simulink model "Implementation_old"  (R2018a)
settings: Solver=ode3  StartTime=0.0  StopTime=50  RelTol=1e-3  EnableMultiTasking=on
values from neighbouring files (symbols this model uses):
  A = [3.3545 -4.3521 2.6058 -0.6082; 1 0 0 0; 0 1 0 0; 0 0 1 0]    [LQGm.m]    (also in Testes_planta.m)
  B = [1;0;0;0]    [LQGm.m]    (also in Testes_planta.m)
  C = [-0.0657 0.1152 0 0]    [LQGm.m]    (also in Testes_planta.m)
  ExtensometerGain = -4.49    [Testes_planta.m]
  Nbar = Nu+K*Nx    [LQGm.m]    (also in Testes_planta.m)
  PotentiometerGain = 33.79    [Testes_planta.m]
undefined symbols (not defined in the file or in its folder): DiscIntNeverNeededParam, K, M, MIO, National_Instruments, PCI
libraries: sldrtlib x2
settings Model: SimulationMode=external  ExtModeTrigDuration=20000  Creator=Alunos  LastModifiedBy=joaj
settings DataIOCC: LimitDataPoints=on  SaveFormat=Array
settings DebuggingCC: LibraryContextMissingDiagnostic=warning  SFUnexpectedBacktrackingDiag=warning  SFNoUnconditionalDefaultTransitionDiag=warning  SFExecutionAtInitializationDiag=none
settings HardwareCC: TargetIntDivRoundTo=Zero  TargetEndianess=LittleEndian  TargetHWDeviceType=Intel->x86/Pentium
settings ModelReferenceCC: PropagateSignalLabelsOutOfModel=off
settings RTWCC: SystemTargetFile=sldrt.tlc  TemplateMakefile=sldrt.tmf  Description=Simulink Desktop Real-Time  RTWCompilerOptimization=on
settings CodeAppCC: MaxIdLength=95  StateflowObjectComments=on
settings SimulinkDesktopRealTimeCC: TargetPreCompLibLocation=C:\Program Files\MATLAB\R2018b\toolbox\sldrt\lib\win64  TargetLangStandard=C89/C90 (ANSI)  SupportVariableSizeSignals=off
settings ConfigComp: CovMetricSettings=dw  CovHtmlReporting=on  CovSaveCumulativeToWorkspaceVar=on  CovSaveSingleToWorkspaceVar=on  CovExternalEMLEnable=off

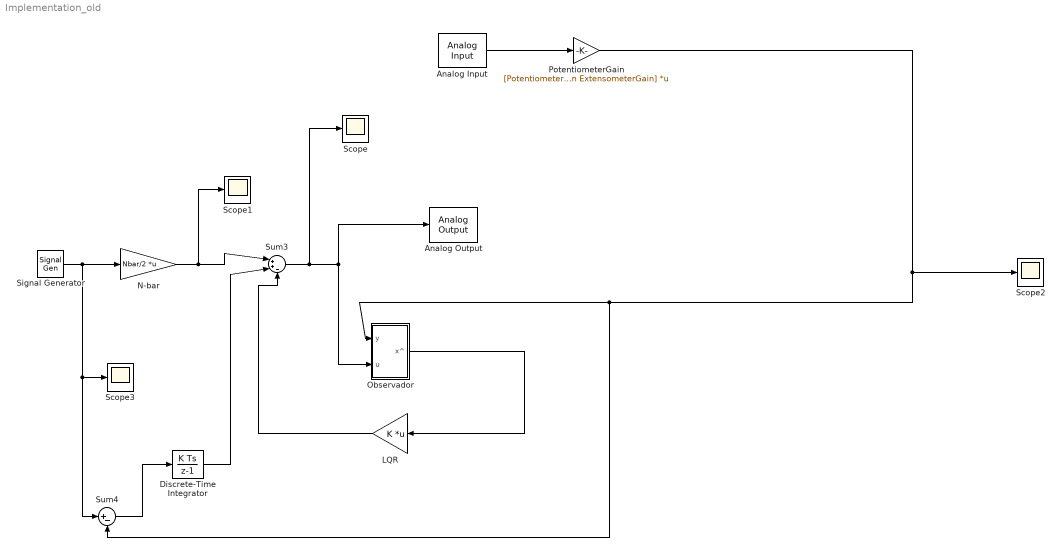
== system Implementation_old ==
  Analog Input : sldrtlib/Analog Input  SampleTime=0.02  MaxMissedTicks=10  ShowMissedTicks=off  YieldWhenWaiting=off  DrvName=National_Instruments/PCI-MIO-16E-4  DrvAddress=4294967295  DrvOptions=[0 0 0 0 0 0]  Channels=[1 2]  RangeMode=1  VoltRange=1  DataType=1
      settings: AttributesFormatString=National Instruments\nPCI-MIO-16E-4 [auto]  SourceProductName=Simulink Desktop Real-Time
  Analog Output : sldrtlib/Analog Output  SampleTime=0.02  MaxMissedTicks=10  ShowMissedTicks=off  YieldWhenWaiting=off  DrvName=National_Instruments/PCI-MIO-16E-4  DrvAddress=4294967295  DrvOptions=[0 0 0 0 0 0]  Channels=1  RangeMode=1  VoltRange=1  InitialValue=0  FinalValue=0
      settings: AttributesFormatString=National Instruments\nPCI-MIO-16E-4 [auto]  SourceProductName=Simulink Desktop Real-Time
  Discrete-Time Integrator : DiscreteIntegrator  gainval=1e-2  ICPrevOutput=DiscIntNeverNeededParam  ICPrevScaledInput=DiscIntNeverNeededParam
  LQR : Gain  Gain=K  Multiplication=Matrix(K*u)
  N-bar : Gain  Gain=Nbar/2  Multiplication=Matrix(K*u)
  Observador : Subsystem
  PotentiometerGain : Gain  Gain=[PotentiometerGain ExtensometerGain]  Multiplication=Matrix(K*u)
  Scope{,1..3} (4 alike) : Scope
  Signal Generator : SignalGenerator  WaveForm=square  Amplitude=30  Frequency=2
  Sum3 : Sum  Inputs=|++-
  Sum4 : Sum  Inputs=|+-
  wires:
  Signal Generator/1 -> Scope3/1, Sum4/1, N-bar/1
  LQR/1 -> Sum3/3
  PotentiometerGain/1 -> Observador/1(y), Sum4/2, Scope2/1
  Observador/1(x^) -> LQR/1
  N-bar/1 -> Sum3/1, Scope1/1
  Sum3/1 -> Scope/1, Analog Output/1, Observador/2(u)
  Sum4/1 -> Discrete-Time Integrator/1
  Discrete-Time Integrator/1 -> Sum3/2
  Analog Input/1 -> PotentiometerGain/1

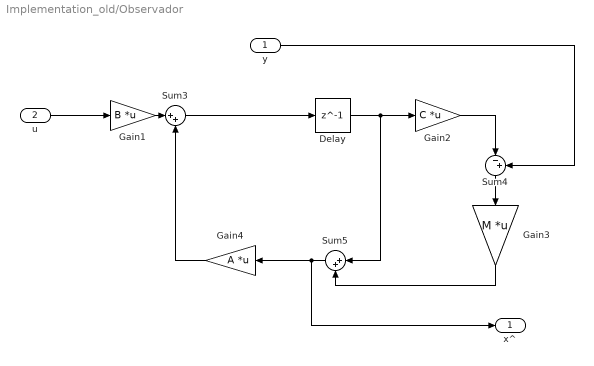
== system Implementation_old/Observador ==
  y : Inport
  u : Inport  Port=2
  Delay : Delay  DelayLength=1  InitialCondition=0
  Gain1 : Gain  Gain=B  Multiplication=Matrix(K*u)
  Gain2 : Gain  Gain=C  Multiplication=Matrix(K*u)
  Gain3 : Gain  Gain=M  Multiplication=Matrix(K*u)
  Gain4 : Gain  Gain=A  Multiplication=Matrix(K*u)
  Sum3 : Sum  Inputs=|++
  Sum4 : Sum  Inputs=|-+
  Sum5 : Sum  Inputs=|++
  x^ : Outport
  wires:
  u/1 -> Gain1/1
  Gain1/1 -> Sum3/1
  Sum4/1 -> Gain3/1
  Gain3/1 -> Sum5/2
  Gain4/1 -> Sum3/2
  Sum5/1 -> x^/1, Gain4/1
  Delay/1 -> Sum5/1, Gain2/1
  Gain2/1 -> Sum4/1
  Sum3/1 -> Delay/1
  y/1 -> Sum4/2
